simulink model "roll_moment_controller"  (R2021b)
settings: Solver=VariableStepAuto  StartTime=0.0  StopTime=10.0  RelTol=1e-3
undefined symbols (not defined in the file): sigbuilder_block
libraries: simulink_extras x1
settings Model: Creator=Ronak Jain  LastModifiedBy=Ronak Jain

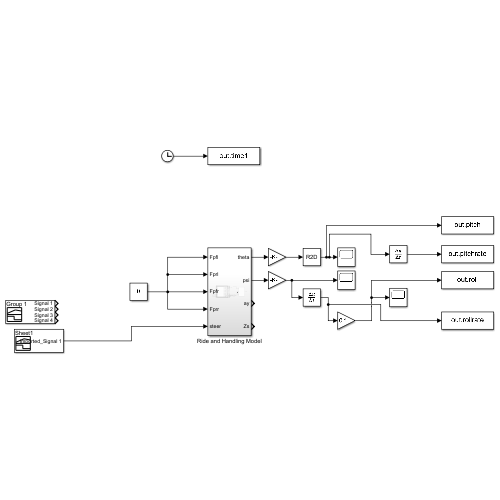
[thumbnail: Simulink's stored preview of the top-level diagram]
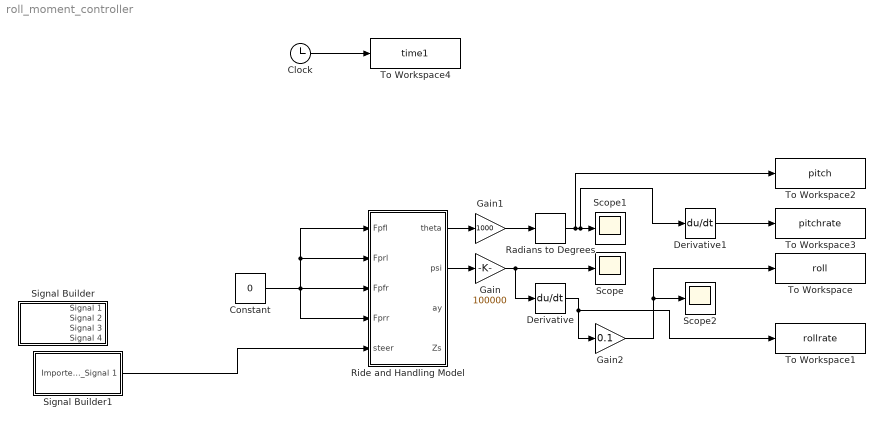
== system roll_moment_controller ==
  Clock : Clock
  Constant : Constant  Value=0
  Derivative : Derivative
  Derivative1 : Derivative
  Gain : Gain  Gain=100000
  Gain1 : Gain  Gain=1000
  Gain2 : Gain  Gain=0.1
  Radians to Degrees : simulink_extras/Transformations/Radians to Degrees
  Ride and Handling Model : Subsystem
  Scope : Scope
  Scope1 : Scope
  Scope2 : Scope
  Signal Builder : Subsystem  Tag=STV Subsys  LoadFcn=sigbuilder_block('load');  StartFcn=sigbuilder_block('start');  StopFcn=sigbuilder_block('stop');  ClipboardFcn=sigbuilder_block('clipboard');  mask(Sigbuilder block){tuvar=[0:10]}
      mask help: Simulink:masks:SigbuilderBlock_MD
      mask init:
      | if ~strcmp(get_param(bdroot(gcbh),'SimulationStatus'),'stopped') tuvar = sigbuilder_block('maskInit'); end
      settings: CopyFcn=sigbuilder_block('copy');  DeleteFcn=sigbuilder_block('delete');  ModelCloseFcn=sigbuilder_block('modelClose');  PreSaveFcn=sigbuilder_block('preSave');  PauseFcn=sigbuilder_block('pause');  ContinueFcn=sigbuilder_block('continue');  NameChangeFcn=sigbuilder_block('namechange');  OpenFcn=sigbuilder_block('open',[5.4 36 1141.2 516.6 ]);  CloseFcn=sigbuilder_block('close');
      mask Display: plot(0, 0, 100, 100,[2, 2, 32, 32, 2], [68, 8, 8, 68, 68],[32, 2], [38, 38], [32, 19, 2],[53, 60, 44], [32, 17, 17, 2],[16, 16, 31, 31]);txt = getActiveGroup(gcbh);text(2, 100, txt,'verticalAlignment', 'top');
  Signal Builder1 : Subsystem  Tag=STV Subsys  LoadFcn=sigbuilder_block('load');  StartFcn=sigbuilder_block('start');  StopFcn=sigbuilder_block('stop');  ClipboardFcn=sigbuilder_block('clipboard');  mask(Sigbuilder block){tuvar=[0:10]}
      mask help: Simulink:masks:SigbuilderBlock_MD
      mask init:
      | if ~strcmp(get_param(bdroot(gcbh),'SimulationStatus'),'stopped') tuvar = sigbuilder_block('maskInit'); end
      settings: CopyFcn=sigbuilder_block('copy');  DeleteFcn=sigbuilder_block('delete');  ModelCloseFcn=sigbuilder_block('modelClose');  PreSaveFcn=sigbuilder_block('preSave');  PauseFcn=sigbuilder_block('pause');  ContinueFcn=sigbuilder_block('continue');  NameChangeFcn=sigbuilder_block('namechange');  OpenFcn=sigbuilder_block('open',[405.6 130.2 550.8 400.2 ]);  CloseFcn=sigbuilder_block('close');
      mask Display: plot(0, 0, 100, 100,[2, 2, 32, 32, 2], [68, 8, 8, 68, 68],[32, 2], [38, 38], [32, 19, 2],[53, 60, 44], [32, 17, 17, 2],[16, 16, 31, 31]);txt = getActiveGroup(gcbh);text(2, 100, txt,'verticalAlignment', 'top');
  To Workspace : ToWorkspace  VariableName=roll  SaveFormat=Timeseries  SampleTime=-1
  To Workspace1 : ToWorkspace  VariableName=rollrate  SaveFormat=Timeseries  SampleTime=-1
  To Workspace2 : ToWorkspace  VariableName=pitch  SaveFormat=Timeseries  SampleTime=-1
  To Workspace3 : ToWorkspace  VariableName=pitchrate  SaveFormat=Timeseries  SampleTime=-1
  To Workspace4 : ToWorkspace  VariableName=time1  SaveFormat=Timeseries  SampleTime=-1
  wires:
  Ride and Handling Model/2(psi) -> Gain/1
  Constant/1 -> Ride and Handling Model/4(Fprr), Ride and Handling Model/3(Fpfr), Ride and Handling Model/1(Fpfl), Ride and Handling Model/2(Fprl)
  Ride and Handling Model/1(theta) -> Gain1/1
  Gain1/1 -> Radians to Degrees/1
  Radians to Degrees/1 -> To Workspace2/1, Derivative1/1, Scope1/1
  Gain/1 -> Derivative/1, Scope/1
  Derivative/1 -> To Workspace1/1, Gain2/1
  Gain2/1 -> To Workspace/1, Scope2/1
  Derivative1/1 -> To Workspace3/1
  Clock/1 -> To Workspace4/1
  Signal Builder1/1(Imported_Signal 1) -> Ride and Handling Model/5(steer)

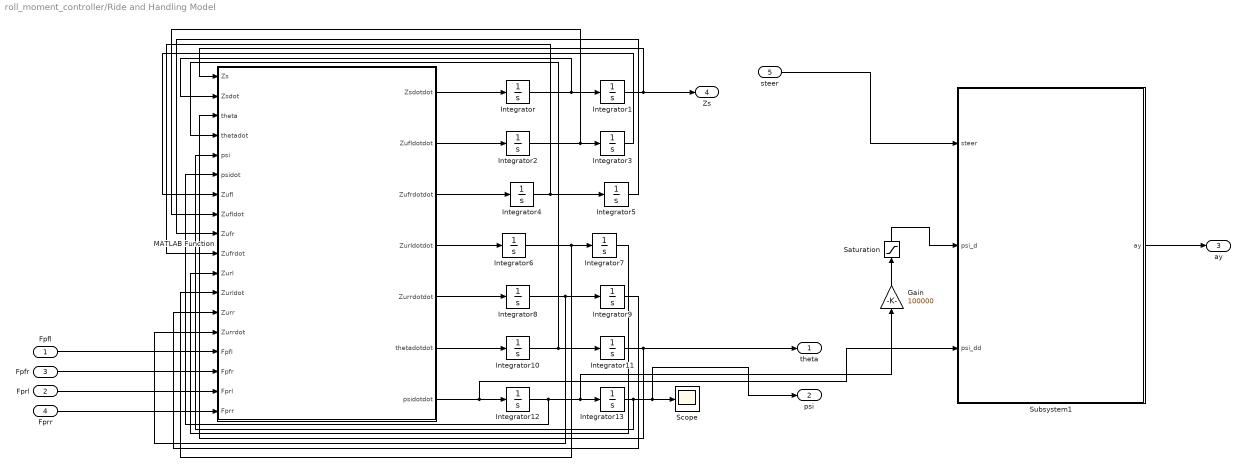
== system roll_moment_controller/Ride and Handling Model ==
  Fpfl : Inport
  Fprl : Inport  Port=2
  Fpfr : Inport  Port=3
  Fprr : Inport  Port=4
  steer : Inport  Port=5
  Gain : Gain  Gain=100000
  Integrator{,1..13} (14 alike) : Integrator  InitialCondition=0.0001
  MATLAB Function : MATLAB Function  TreatAsAtomicUnit=on
  Saturation : Saturate  UpperLimit=10  LowerLimit=-1
  Scope : Scope
  Subsystem1 : Subsystem
  theta : Outport
  psi : Outport  Port=2
  ay : Outport  Port=3
  Zs : Outport  Port=4
  wires:
  MATLAB Function/7(psidotdot) -> Subsystem1/3(psi_dd), Integrator12/1
  MATLAB Function/1(Zsdotdot) -> Integrator/1
  Integrator8/1 -> MATLAB Function/14(Zurrdot), Integrator9/1
  MATLAB Function/3(Zufrdotdot) -> Integrator4/1
  Integrator13/1 -> psi/1, Scope/1, MATLAB Function/5(psi)
  MATLAB Function/6(thetadotdot) -> Integrator10/1
  Integrator2/1 -> MATLAB Function/8(Zufldot), Integrator3/1
  Integrator6/1 -> MATLAB Function/12(Zurldot), Integrator7/1
  Integrator4/1 -> MATLAB Function/10(Zufrdot), Integrator5/1
  Integrator/1 -> MATLAB Function/2(Zsdot), Integrator1/1
  Integrator5/1 -> MATLAB Function/9(Zufr)
  Integrator11/1 -> theta/1, MATLAB Function/3(theta)
  Integrator10/1 -> MATLAB Function/4(thetadot), Integrator11/1
  Integrator1/1 -> Zs/1, MATLAB Function/1(Zs)
  Integrator12/1 -> Gain/1, Integrator13/1, MATLAB Function/6(psidot)
  Fpfr/1 -> MATLAB Function/16(Fpfr)
  Integrator9/1 -> MATLAB Function/13(Zurr)
  MATLAB Function/2(Zufldotdot) -> Integrator2/1
  MATLAB Function/5(Zurrdotdot) -> Integrator8/1
  Integrator3/1 -> MATLAB Function/7(Zufl)
  MATLAB Function/4(Zurldotdot) -> Integrator6/1
  Integrator7/1 -> MATLAB Function/11(Zurl)
  Fprl/1 -> MATLAB Function/17(Fprl)
  Fpfl/1 -> MATLAB Function/15(Fpfl)
  Fprr/1 -> MATLAB Function/18(Fprr)
  steer/1 -> Subsystem1/1(steer)
  Subsystem1/1(ay) -> ay/1
  Gain/1 -> Saturation/1
  Saturation/1 -> Subsystem1/2(psi_d)

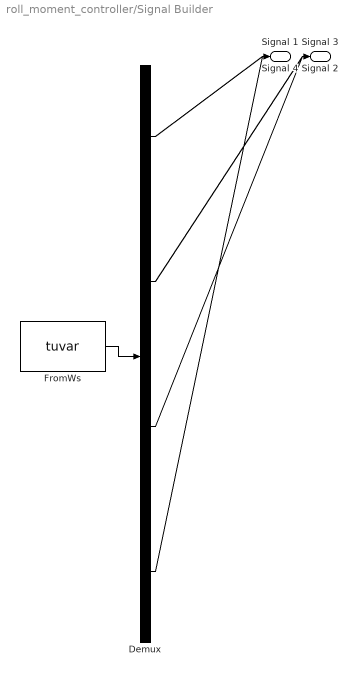
== system roll_moment_controller/Signal Builder ==
  Demux : Demux  Tag=STV Demux
      settings: DisplayOption=none
  FromWs : FromWorkspace  Tag=STV FromWs  VariableName=tuvar
      SigBuilderData=|
      | common.afterFinalStr = 'Extrapolate'
      | common.sampleTime = 0
      | dataSet.timeRange = [0 10]
      | dataSet.name = 'Group 1'
      | sbobj.Groups.Name = 'Group 1'
      | sbobj.Groups.Signals(1).Name = 'Signal 1'
      | sbobj.Groups.Signals(1).XData = [0 4 4 6 6 10]
      | sbobj.Groups.Signals(1).YData = [0 0.125 1 1 0 0]
      | sbobj.Groups.Signals(2).Name = 'Signal 2'
      | sbobj.Groups.Signals(2).XData = [0 10]
      | sbobj.Groups.Signals(2).YData = [1 1]
      | sbobj.Groups.Signals(3).Name = 'Signal 3'
      | sbobj.Groups.Signals(3).XData = [0 0.125 0.25 0.375 0.5 0.625 0.75 0.875 1 1.125 1.25 1.375 1.5 1.625 1.75 1.875 2 2.125 2.25 2.375 2.5 2.625 2.75 2.875 3 3.125 3.25 3.375 3.5 3.625 3.75 3.875 4 4.125 4.25 4.375 4.5 4.625 4.75 4.875 5 5.125 5.25 5.375 5.5 5.625 5.75 5.875 6 6.125 6.25 6.375 6.5 6.625 6.75 6.875 7 7.125 7.25 7.375 7.5 7.625 7.75 7.875 8 8.125 8.25 8.375 8.5 8.625 8.75 8.875 9 9.125 9.25 9.375 9.5 9.625 9.75 9.875 10]
      | sbobj.Groups.Signals(3).YData = [1 29.2842712475 41 29.2842712475 1 -27.2842712475 -39 -27.2842712475 1 29.2842712475 41 29.2842712475 1 -27.2842712475 -39 -27.2842712475 1 29.2842712475 41 29.2842712475 1 -27.2842712475 -39 -27.2842712475 1 29.2842712475 41 29.2842712475 1 -27.2842712475 -39 -27.2842712475 1 29.2842712475 41 29.2842712475 1 -27.2842712475 -39 -27.2842712475 1 29.2842712475 41 29.2842712475 1 -27.2842712475 -39 -27.2842712475 1 29.2842712475 41 29.2842712475 1 -27.2842712475 -39 -27.2842712475 1 29.2842712475 41 29.2842712475 1 -27.2842712475 -39 -27.2842712475 1 29.2842712475 41 29.2842712475 1 -27.2842712475 -39 -27.2842712475 1 29.2842712475 41 29.2842712475 1 -27.2842712475 -39 -27.2842712475 1]
      | sbobj.Groups.Signals(4).Name = 'Signal 4'
      | sbobj.Groups.Signals(4).XData = [0 1.25 2.5 3.75 5 6.25 7.5 8.75 10]
      | sbobj.Groups.Signals(4).YData = [1 29.2842712475 41 29.2842712475 1 -27.2842712475 -27 -27.2842712475 1]
  Signal 1 : Outport  Tag=STV Outport
  Signal 2 : Outport  Tag=STV Outport  Port=2
  Signal 3 : Outport  Tag=STV Outport  Port=3
  Signal 4 : Outport  Tag=STV Outport  Port=4
  wires:
  FromWs/1 -> Demux/1
  Demux/1 -> Signal 1/1
  Demux/2 -> Signal 2/1
  Demux/3 -> Signal 3/1
  Demux/4 -> Signal 4/1

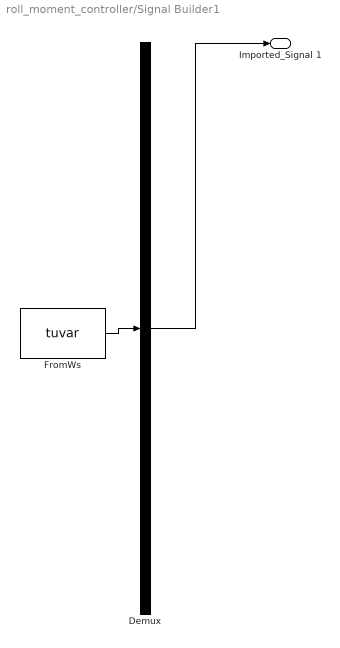
== system roll_moment_controller/Signal Builder1 ==
  Demux : Demux  Tag=STV Demux  Outputs=1
      settings: DisplayOption=none
  FromWs : FromWorkspace  Tag=STV FromWs  VariableName=tuvar
      SigBuilderData=|
      | common.afterFinalStr = 'Extrapolate'
      | common.sampleTime = 0
      | dataSet.timeRange = [0 10]
      | dataSet.name = 'Sheet1'
      | sbobj.Groups.Name = 'Sheet1'
      | sbobj.Groups.Signals.Name = 'Imported_Signal 1'
      | sbobj.Groups.Signals.XData = [0 0.0200400801603 0.0400801603206 0.060120240481 0.0801603206413 0.100200400802 0.120240480962 0.140280561122 0.160320641283 0.180360721443 0.200400801603 0.220440881764 ... (500 elements, 1x500)]
      | sbobj.Groups.Signals.YData = [0 0 0 0 0 0 0 0 0 0 0 0 0 0 0 0 0 0 0 0 0 0 0 0 0 0 0 0 0 0 0 0 0 0 0 0 0 0 0 0 0 0 0 0 0 0 0 0 0 0 0 0 0 0 0 0 0 0 0 0 0 0 0 0 0 0 0 0 0 0 0 0 0 0 0 0 0 0 0 0 0 0 0 0 0 0 0 0 0 0 0 0 0 0 0 0 0 0 0 0 0 0 0 0 0 0 0 0 0 0 0 0 0 0 0 0 0 0 0 0 0 0 0 0 0 0 0 0 0 0 0 0 0 0 0 0 0 0 0 0 0 0 0 0 0 0 0 0 0 0 4.32865731463 18.7575150301 33.1863727455 45 45 45 45 45 45 45 45 45 45 45 45 45 45 45 45 45 45 45 45 45 45 45 45 45 45 45 45 32.376753507 17.9478957916 3.51903807615 -10.9098196393 -25.3386773547 -39.7675350701 -45 -45 -45 -45 -45 -45 -45 -45 -45 -45 -45 -45 -45 -45 -45 -45 -45 -45 -45 -45 -45 -45 -45 -45 -45 -45 -45 -45 -45 -45 -45 -45 -45 -45 -45 -45 -45 -45 -45 -45 -45 -45 -45 -45 -45 -45 -45 -45 -45 -45 -45 -45 -45 -45 -45 -45 -45 -45 -45 -45 -45 -45 -45 -45 -45 -45 -45 -45 -45 -45 -45 -45 -45 -45 -45 -45 -45 -45 -45 -45 -45 -45 -45 -45 -45 -45 -45 -45 -45 -45 -45 -45 -45 -45 -45 -45 -45 -45 -45 -45 -45 -45 -45 -45 -45 -45 -45 -45 -45 -45 -45 -45 -45 -45 -45 -45 -45 -45 -45 -45 -45 -45 -45 -45 -45 -45 -45 -45 -45 -45 -45 -45 -45 -45 -45 -45 -45 -45 -45 -45 -45 -45 -45 -45 -45 -45 -45 -45 -45 -41.9038076152 -27.4749498998 -13.0460921844 0 0 0 0 0 0 0 0 0 0 0 0 0 0 0 0 0 0 0 0 0 0 0 0 0 0 0 0 0 0 0 0 0 0 0 0 0 0 0 0 0 0 0 0 0 0 0 0 0 0 0 0 0 0 0 0 0 0 0 0 0 0 0 0 0 0 0 0 0 0 0 0 0 0 0 0 0 0 0 0 0 0 0 0 0 0 0 0 0 0 0 0 0 0 0 0 0 0 0 0 0 0 0 0 0 0 0 0 0 0 0 0 0 0 0 0 0 0 0 0 0 0 0 0 0 0 0 0 0 0 0 0 0 0 0 0 0 0 0 0 0 0 0 0 0 0 0 0 0 0 0 0 0 0 0 0 0 0 0 0 0]
  Imported_Signal 1 : Outport  Tag=STV Outport
  wires:
  Demux/1 -> Imported_Signal 1/1
  FromWs/1 -> Demux/1

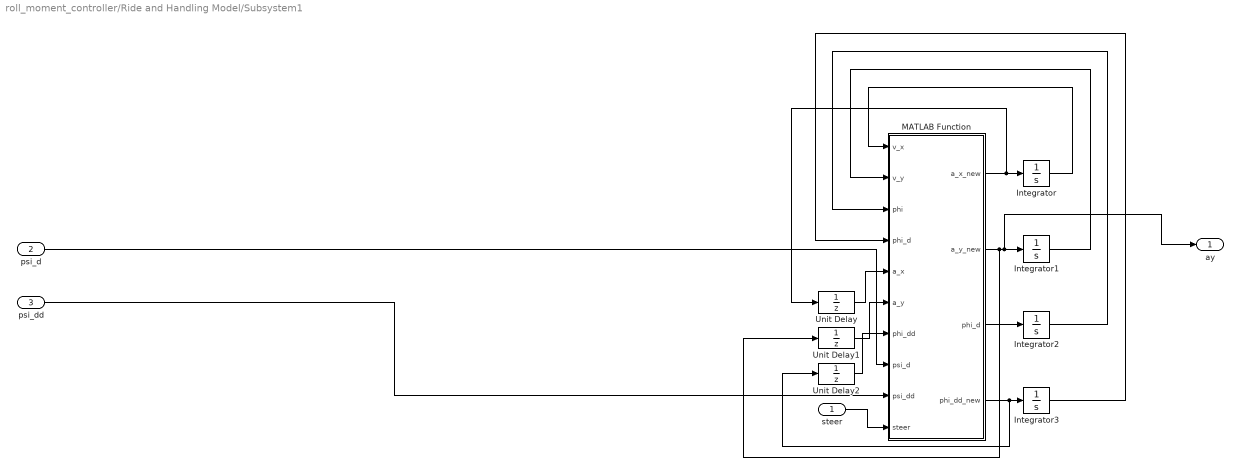
== system roll_moment_controller/Ride and Handling Model/Subsystem1 ==
  steer : Inport
  psi_d : Inport  Port=2
  psi_dd : Inport  Port=3
  Integrator{,1..3} (4 alike) : Integrator  InitialCondition=0.0001
  MATLAB Function : MATLAB Function  TreatAsAtomicUnit=on
  Unit Delay : UnitDelay  SampleTime=-1  HasFrameUpgradeWarning=on
  Unit Delay1 : UnitDelay  SampleTime=-1  HasFrameUpgradeWarning=on
  Unit Delay2 : UnitDelay  SampleTime=-1  HasFrameUpgradeWarning=on
  ay : Outport
  wires:
  MATLAB Function/1(a_x_new) -> Unit Delay/1, Integrator/1
  Integrator/1 -> MATLAB Function/1(v_x)
  MATLAB Function/2(a_y_new) -> Unit Delay1/1, ay/1, Integrator1/1
  Integrator1/1 -> MATLAB Function/2(v_y)
  MATLAB Function/3(phi_d) -> Integrator2/1
  Integrator2/1 -> MATLAB Function/3(phi)
  MATLAB Function/4(phi_dd_new) -> Unit Delay2/1, Integrator3/1
  Integrator3/1 -> MATLAB Function/4("phi_d ")
  Unit Delay/1 -> MATLAB Function/5(a_x)
  Unit Delay1/1 -> MATLAB Function/6(a_y)
  Unit Delay2/1 -> MATLAB Function/7(phi_dd)
  steer/1 -> MATLAB Function/10(steer)
  psi_d/1 -> MATLAB Function/8(psi_d)
  psi_dd/1 -> MATLAB Function/9(psi_dd)

== matlab function roll_moment_controller/Ride and Handling Model/MATLAB Function ==
  data: Zs input; Zsdotdot output; Zsdot input; theta input; thetadot input; psi input; psidot input; Zufl input; Zufldot input; Zufr input; Zufrdot input; Zurl input; Zurldot input; Zurr input; Zurrdot input; Fpfl input; Fpfr input; Fprl input; Fprr input; Zufldotdot output; Zufrdotdot output; Zurldotdot output; Zurrdotdot output; thetadotdot output; psidotdot output
function [Zsdotdot,Zufldotdot, Zufrdotdot, Zurldotdot, Zurrdotdot, thetadotdot, psidotdot] = ...
    fcn(Zs,Zsdot,theta,thetadot,psi,psidot,Zufl,Zufldot,Zufr, Zufrdot,Zurl, Zurldot,...
    Zurr, Zurrdot,Fpfl,Fpfr,Fprl,Fprr)

Iyy = 2498.900;
Ixx = 440.911;
w = 1.54;
Ksf = 30000; %N/mm
Ksr = 30000; %N/mm
Csf = 750;
Csr = 750;
lf = 1.01476;
lr = 1.67524;
M = 1704;
M_uf = 98.1;
M_ur = 79.7;
g = 9.81;
phi_ss_ay = (4*pi)/(180*9.81);
M_s = M - M_uf - M_ur;
h_f = 0.130;
h_r = 0.110;
h_cgs = 0.567851;
L = lf + lr;
h_o = h_f + lf*(h_r - h_f)/L;
h_s = h_cgs - h_o;

k_t = (M_s * h_s)/(phi_ss_ay) +M*g*h_s;

Zsdotdot = (-2*(Ksf + Ksr)*Zs - 2*(Csf + Csr)*Zsdot + 2*(lf*Ksf - lr*Ksr)*theta ...
    +2*(lf*Csf - lr*Csr)*thetadot + Ksf*Zufl + Csf*Zufldot + Ksf*Zufr + Csf*Zufrdot+...
    Ksr*Zurl + Csr*Zurldot + Ksr*Zurr + Csr*Zurrdot + Fpfl + Fpfr + Fprl + Fprr)/M;

Zufldotdot = (Ksf*Zs + Csf*Zsdot - lf*Ksf*theta - lf*Csf*thetadot+ 0.5*w*Ksf*psi+...
    0.5*w*Csf*psidot - (Ksf + k_t)*Zufl - Csf*Zufldot - Fpfl)/M;


Zufrdotdot = (Ksf*Zs + Csf*Zsdot - lf*Ksf*theta - lf*Csf*thetadot - 0.5*w*Ksf*psi...
    - 0.5*w*Csf*psidot - (Ksf+k_t)*Zufr - Csf*Zufrdot  - Fpfr)/M;

Zurldotdot = (Ksr*Zs + Csr*Zsdot + lr*Ksr*theta + lr*Csr*thetadot + 0.5*w*Ksr*psi + ...
    0.5*w*Csr*psidot - (Ksr + k_t)*Zurl - Csr*Zurldot  - Fprl)/M;

Zurrdotdot = (Ksr*Zs + Csr*Zsdot + lr*Ksr*theta + lr*Csr*thetadot - 0.5*w*Ksr*psi - ...
    0.5*w*Csr*psidot - (Ksr + k_t)*Zurr - Csr*Zurrdot  - Fprr)/M;

thetadotdot = (2*(lf*Ksf - lr*Ksr)*Zs + 2*(lf*Csf - lr*Csr)*Zsdot - 2*((lf^2)*Ksf + (lr^2)*Ksr)*theta - ...
    2*((lf^2)*Csf + (lr^2)*Csr)*thetadot - lf*Ksf*Zufl - lf*Csf*Zufldot - lf*Ksf*Zufr - ...
    lf*Csf*Zufrdot + lr*Ksr*Zurl + lr*Csr*Zurldot + lr*Ksr*Zurr + lr*Csr*Zurrdot - ...
    (Fpfl + Fpfr)*lf + (Fprl + Fprr)*lr)/Iyy;

psidotdot = (-0.5*(w^2)*(Ksf+Ksr)*psi + -0.5*(w^2)*(Csf+Csr)*psidot + 0.5*w*Ksf*Zufl + ...
    0.5*w*Csf*Zufldot - 0.5*w*Ksf*Zufr - 0.5*w*Csf*Zufrdot + 0.5*w*Ksr*Zurl + ...
    0.5*w*Csr*Zurldot - 0.5*w*Ksr*Zurr - 0.5*w*Csr*Zurrdot + (Fpfl + Fprl)*(w/2) - (Fpfr + Fprr)*(w/2))/Ixx;

end

== matlab function roll_moment_controller/Ride and Handling Model/Subsystem1/MATLAB Function ==
  data: v_x input; a_x_new output; v_y input; phi input; phi_d input; a_x input; a_y input; phi_dd input; psi_d input; psi_dd input; steer input; a_y_new output; phi_d output; phi_dd_new output
function [a_x_new, a_y_new, phi_d, phi_dd_new] = ...
    fcn(v_x, v_y,phi, phi_d,a_x,a_y,phi_dd,psi_d,psi_dd,steer)

%==constants==%
g = 9.81;

%------------------%
%Car physical variables
l_fs = 1.01476;
l_rs = 1.67524;
t_f = 1.540;
t_r = 1.530;
h_f = 0.130;
h_r = 0.110;
h_cgs = 0.567851;
h_cguf = 0.320;
h_cgur = 0.320;
M = 1704.7;
M_uf = 98.1;
M_ur = 79.7;
I_xxs = 440.911;
I_xys = 0;
I_xzs = 7.54097;
I_yys = 2498.900;
I_yzs = 0;
I_zzs = 2619.28;
I_zzuf = M_uf*(t_f/2)^2;
I_zzur = M_ur*(t_r/2)^2;
I_tlf = 0.99;
I_trf = 0.99;
I_tlr = 0.99;
I_trr = 0.99;
%spring/dampers
K_spf = 30000; %N/mm
K_spr = 30000; %N/mm
B_f = 299.15; %N-s/mm
B_r = 299.15; %N-s/mm
%anti_roll bars
K_rf = 384.0*180/pi; %Nm/rad
K_rr = 344.4*180/pi;
%roll stiffness
K_phif = 0.766*K_spf*1000*t_f^2/2 + K_rf;%
K_phir = 0.827*K_spr*1000*t_r^2/2 + K_rr;%
K_phi = (K_phif + K_phir);
%roll damping
B_phif = 0.766*B_f*1000*t_f^2/2; %Nm-s/rad
B_phir = 0.827*B_r*1000*t_r^2/2;
B_phi = (B_phif + B_phir);
K_sr = 15.97; %steering-to-wheel angle ratio
%==calculated parameters==%
L = l_fs + l_rs;
M_s = M - M_uf - M_ur;
l_cgs = (M_ur*l_rs - M_uf*l_fs)/M;
l_f = l_fs + l_cgs;
l_r = l_rs - l_cgs;
M_f = M*l_r/L;
M_r = M*l_f/L;
h_o = h_f + l_f*(h_r - h_f)/L;
h_s = h_cgs - h_o;
h_uf = h_cguf - h_o;
h_ur = h_cgur - h_o;
h_cg = (M_s*h_cgs + M_uf*h_cguf + M_ur*h_cgur)/M;
%----------------------------%
%==tire properties==%
varx = [... 
    0.0, 0.0;... 
    0.1, 0.6;... 
    0.15, 0.85;... 
    1.0, 0.4]; %slip curve coordinates (slip-%, mu)
vary = [... 
    0.0, 0.0;... 
    0.08, 0.4;... 
    0.15, 0.6;... 
    0.3, 0.8;... 
    1.0, 0.4]; %slip curve coordinates (slip-%, mu)
varM = [... 
    0.0, 0.0;...
    0.1, 0.0005;...
    0.3, 0.00025;... 
    1.0, 0.0]; %slip angle (slip-angle, Moment-arm)
%tire properties
t_wid = 0.175;
t_rad = 0.292;
t_pressure = 275000;
%---------------------%
%==steering inputs==%
d_steer = steer;
%-------------------%
%==calculate internal accelerations==%
a_sx = a_x ...
    - psi_d*v_y ...
    - 2*h_s*phi_d*psi_d*cos(phi) ...
    - l_cgs*psi_d^2;
a_sy = psi_d*v_x + l_cgs*psi_dd + h_s*cos(phi)*phi_dd - h_s*phi_d^2*sin(phi) - h_s*psi_d^2*sin(phi);
a_ufx = a_x - l_f*psi_d^2;
a_ufy = a_y + l_f*psi_dd;
a_urx = a_x + l_r*psi_d^2;
a_ury = a_y - l_r*psi_dd;
%-------------------------------------%
%==rotation Matrix==%
ROT = [1,0,0; 
    0,cos(phi),sin(phi); 
    0,-sin(phi),cos(phi)];
I_b = [I_xxs+M_s*h_s^2,I_xys,I_xzs+M_s*h_s*l_cgs;... 
    I_xys,I_yys+M_s*(h_s^2+l_cgs^2),I_yzs;... 
    I_xzs+M_s*h_s*l_cgs,I_yzs,I_zzs+M_s*l_cgs^2];
I_c = ROT*I_b*ROT'; %chassis M.o.I. tensor
I_zzus = M_uf*l_f^2 + ... 
    M_ur*l_r^2 + ... 
    I_zzuf + I_zzur;
I_xxo = I_c(1,1);
I_zzo = I_c(3,3) + I_zzus; %effective I_zz
%---------------------------------------------%
%==Dynamic Weight Transfer Forces==%
Fzax = (M_s*h_s*a_sx + M_uf*h_uf*a_ufx + M_ur*h_ur*a_urx)/(2*L);
Fzayf = 1/t_f*(M_s*l_r*h_f/L*a_sy + M_uf*h_uf*a_ufy);
Fzayr = 1/t_r*(M_s*l_f*h_r/L*a_sy + M_ur*h_ur*a_ury);
Fzphif = -1/t_f*(K_phif*phi + B_phif*phi_d);
Fzphir = -1/t_r*(K_phir*phi + B_phir*phi_d);
%----------------------------------%
%==Tire Normal Forces==%
Fzlf = M*g*l_r/(2*L) - Fzax - Fzayf + Fzphif;
Fzrf = M*g*l_r/(2*L) - Fzax + Fzayf - Fzphif;
Fzlr = M*g*l_f/(2*L) + Fzax - Fzayr + Fzphir;
Fzrr = M*g*l_f/(2*L) + Fzax + Fzayr - Fzphir;
%----------------------%
%==Tire Longitudinal/Lateral Forces==%
%left front wheel velocity
v_xlf = v_x + psi_d*t_f/2;
v_ylf = v_y + psi_d*l_f;
%right front wheel velocity
v_xrf = v_x - psi_d*t_f/2;
v_yrf = v_y + psi_d*l_f;
%left rear wheel velocity
v_xlr = v_x + psi_d*t_r/2;
v_ylr = v_y - psi_d*l_r;
%right rear wheel velocity
v_xrr = v_x - psi_d*t_r/2;
v_yrr = v_y - psi_d*l_r;
%tire updates
omega_lf = (v_xlf^2 + v_ylf^2)^(1/2);
omega_rf = (v_xrf^2 + v_yrf^2)^(1/2);
omega_lr = (v_xlr^2 + v_ylr^2)^(1/2);
omega_rr = (v_xrr^2 + v_yrr^2)^(1/2);
%==Linear Cruise Control=%
if v_x < 11.1
    if omega_lf > omega_rf
        Mtlf = (11.1 - v_x)*200;
        Mtrf = 0;
    else
        Mtlf = 0;
        Mtrf = (11.1 - v_x)*200;
    end
else
    Mtlf = 0;
    Mtrf = 0;
end
Mtlf = 0;
Mtrf = 0;
Mtlr = 0;
Mtrr = 0;
%-------------------------%
%get steering angle
delta = d_steer/(180*K_sr)*pi; %radians
beta = atan(v_y/v_x);
beta_lf = atan(v_ylf/v_xlf);
beta_rf = atan(v_yrf/v_xrf);
beta_lr = atan(v_ylr/v_xlr);
beta_rr = atan(v_yrr/v_xrr);
%Interpolate forces
%Linearized Force Coefficients (C_alpha)
C_alf = vary(2,2)/vary(2,1)*Fzlf;
C_arf = vary(2,2)/vary(2,1)*Fzrf;
C_alr = vary(2,2)/vary(2,1)*Fzlr;
C_arr = vary(2,2)/vary(2,1)*Fzrr;
a_lf = beta_lf - delta;
a_rf = beta_rf - delta;
a_lr = beta_lr;
a_rr = beta_rr;
%Linear Cruise Control for constant v_x
if v_x < 11.1
    Fxtf = (11.1-v_x)*20000;
else
    Fxtf = 0; %no torque
end
Fxtlf = 0;
Fxtrf = 0;
Fxtlr = 0;
Fxtrr = 0;
Fytlf = -a_lf*C_alf;
Fytrf = -a_rf*C_arf;
Fytlr = -a_lr*C_alr;
Fytrr = -a_rr*C_arr;
Fxlf = Fxtlf*cos(delta) - Fytlf*sin(delta);
Fxrf = Fxtrf*cos(delta) - Fytrf*sin(delta);
Fxlr = Fxtlr;
Fxrr = Fxtrr;
Fylf = Fytlf*cos(delta) + Fxtlf*sin(delta);
Fyrf = Fytrf*cos(delta) + Fxtrf*sin(delta);
Fylr = Fytlr;
Fyrr = Fytrr;
Mzlf = 0;
Mzrf = 0;
Mzlr = 0;
Mzrr = 0;
%---------------------------------------%
%Omeaga/Alpha of Wheels
%==Torques==%
T_phif = -K_phif*phi - B_phif*phi_d;
T_phir = -K_phir*phi - B_phir*phi_d;
%-----------%
%==Sum forces and torques==%
sigFx = Fxlf + Fxrf + Fxlr + Fxrr;
sigFy = Fylf + Fyrf + Fylr + Fyrr;
sigTxs = T_phif + T_phir - ... 
    M_s*g*h_s*sin(phi) + M_s*h_s*a_sy*cos(phi);

%--------------------------%

%==Update independent variables==%
a_x_new = (sigFx + ... 
    M_s.*(-2*h_s.*phi_d.*psi_d.*cos(phi) - ... 
    h_s.*psi_dd.*sin(phi)))./M;
a_y_new = (sigFy - ... 
    M_s*(-h_s*phi_dd*cos(phi) + ... 
    h_s*phi_d^2*sin(phi) + ... 
    h_s*psi_d^2*sin(phi)))./M;
phi_dd_new = (sigTxs - ... 
    (I_xzs+M_s*h_s*l_cgs)*cos(phi)*psi_dd + ... 
    (I_xzs+M_s*h_s*l_cgs)*sin(phi)*phi_d*psi_d + ... 
    (I_zzs - I_yys - M_s*h_s^2)*sin(phi)*cos(phi)*psi_d^2)./ ... 
    (I_xxs+M_s*h_s^2);
%X
end
